simulink model "vschvdc"  (R2023a)
settings: Solver=ode45  StartTime=0.0  StopTime=10.0  RelTol=1e-3
InitFcn:
  | P=1e6;
  | V=6e3;
  | F=50;
  | 
  | VDC=6e3;
  | C=200e-6;
  | 
  | R=1e-3;
  | L=0.1;
  | Ts_control=50e-6;
  | Ts=1e-6;
undefined symbols (not defined in the file): D1, Delta, DiscIntNeverNeededParam, init, Ki, Kp, LOW, UP
libraries: spsThreePhaseVIMeasurementLib x6, spsGroundLib x2, spsabctodq0Lib x2, spsThreePhaseSeriesRLCBranchLib x2, spsThreePhaseSeriesRLCLoadLib x2, spsThreePhaseTransformerTwoWindingsLib x2, spsSeriesRLCBranchLib x2, spsUniversalBridgeLib x2, spsVoltageMeasurementLib x2, spsPiSectionLineLib x2, spsThreePhaseMutualInductanceZ1Z0Lib x2, spsThreePhaseProgrammableVoltageSourceLib x2
settings Model: Creator=11094  LastModifiedBy=11094

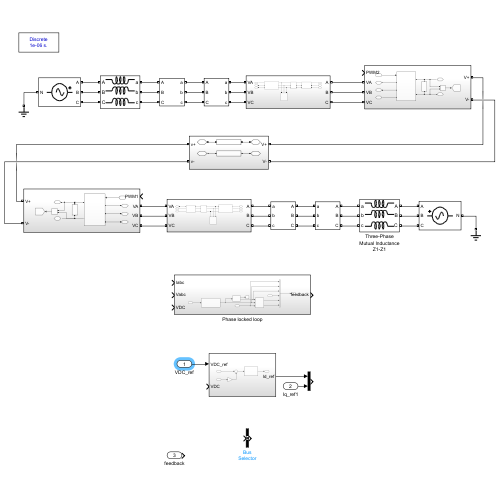
[thumbnail: Simulink's stored preview of the top-level diagram]
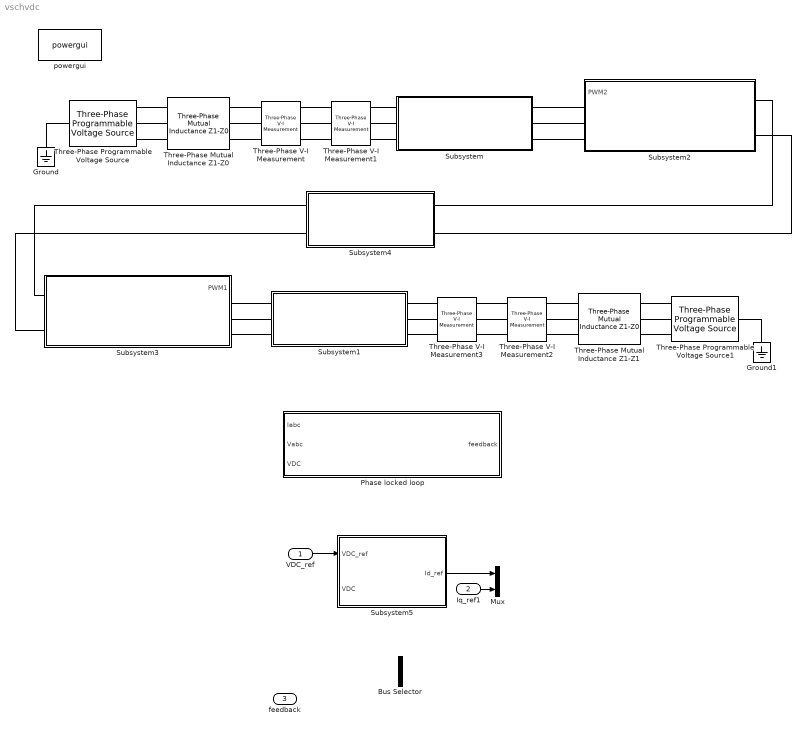
== system vschvdc ==
  VDC_ref : Inport
  Iq_ref1 : Inport  Port=2
  feedback : Inport  Port=3
  Bus Selector : BusSelector  OutputSignals=signal1
  Ground : spsGroundLib/Ground  LConnTagsString=a
  Ground1 : spsGroundLib/Ground  LConnTagsString=a
  Mux : Mux  Inputs=2
  Phase locked loop : Subsystem
  Subsystem : Subsystem
  Subsystem1 : Subsystem
  Subsystem2 : Subsystem
  Subsystem3 : Subsystem
  Subsystem4 : Subsystem
  Subsystem5 : Subsystem
  Three-Phase Mutual Inductance Z1-Z0 : spsThreePhaseMutualInductanceZ1Z0Lib/Three-Phase Mutual Inductance Z1-Z0  LConnTagsString=a|b|c  RConnTagsString=A|B|C  PositiveSequence="[ 220e3^2/(10*P)/10  220e3^2/(10*P)/(2*pi*50)]"  ZeroSequence="[ 220e3^2/(10*P)/10*3  220e3^2/(10*P)/(2*pi*50)*3]"
      settings: AttributesFormatString=\n
      settings: LibrarySourceBlock=|
      | sps_lib/Power Grid Elements/Three-Phase
      | Mutual Inductance
      | Z1-Z0
  Three-Phase Mutual Inductance Z1-Z1 : spsThreePhaseMutualInductanceZ1Z0Lib/Three-Phase Mutual Inductance Z1-Z0  LConnTagsString=a|b|c  RConnTagsString=A|B|C  PositiveSequence="[ 220e3^2/(10*P)/10  220e3^2/(10*P)/(2*pi*50)]"  ZeroSequence="[ 220e3^2/(10*P)/10*3  220e3^2/(10*P)/(2*pi*50)*3]"
      settings: AttributesFormatString=\n
      settings: LibrarySourceBlock=|
      | sps_lib/Power Grid Elements/Three-Phase
      | Mutual Inductance
      | Z1-Z0
  Three-Phase Programmable Voltage Source : spsThreePhaseProgrammableVoltageSourceLib/Three-Phase Programmable Voltage Source  PositiveSequence="[220e3  0 50]"  VariationEntity=None  VariationType=Table of time-amplitude pairs  VariationTypeAlt=Step  VariationStep=0.5  VariationRate=10  VariationMagnitude=0.3  VariationFrequency=2  VariationTiming=[1 2]  VariationPhaseA=off  Amplitudes=[1 0.8 1.2 1.0]  TimeValues=[0 0.1 0.15 0.2]  HarmonicGeneration=off  HarmonicA=[3 0.2 -25 0]  HarmonicB=[2 0.15 35 2]  Timing="[0.05  3]"  BusType=swing  Pref=0  Qref=0  Qmin=-inf  Qmax=inf
  Three-Phase Programmable Voltage Source1 : spsThreePhaseProgrammableVoltageSourceLib/Three-Phase Programmable Voltage Source  PositiveSequence="[220e3  0 50]"  VariationEntity=None  VariationType=Table of time-amplitude pairs  VariationTypeAlt=Step  VariationStep=0.5  VariationRate=10  VariationMagnitude=0.3  VariationFrequency=2  VariationTiming=[1 2]  VariationPhaseA=off  Amplitudes=[1 0.8 1.2 1.0]  TimeValues=[0 0.1 0.15 0.2]  HarmonicGeneration=off  HarmonicA=[3 0.2 -25 0]  HarmonicB=[2 0.15 35 2]  Timing="[0.05  3]"  BusType=swing  Pref=0  Qref=0  Qmin=-inf  Qmax=inf
  Three-Phase V-I Measurement : spsThreePhaseVIMeasurementLib/Three-Phase V-I Measurement  VoltageMeasurement=phase-to-phase  SetLabelV=on  LabelV=Vabc2  Vpu=off  VpuLL=off  CurrentMeasurement=yes  SetLabelI=on  LabelI=Iabc2  Ipu=off  Pbase=100e6  Vbase=500e3  OutputType=Complex  PhasorSimulation=off  PSBequivalent=0
  Three-Phase V-I Measurement1 : spsThreePhaseVIMeasurementLib/Three-Phase V-I Measurement  VoltageMeasurement=phase-to-phase  SetLabelV=on  LabelV=Vabc_B3  Vpu=off  VpuLL=on  CurrentMeasurement=yes  SetLabelI=on  LabelI=Iabc_B3  Ipu=on  Pbase=P  Vbase=V  OutputType=Complex  PhasorSimulation=off  PSBequivalent=0
  Three-Phase V-I Measurement2 : spsThreePhaseVIMeasurementLib/Three-Phase V-I Measurement  VoltageMeasurement=phase-to-phase  SetLabelV=on  LabelV=Vabc1  Vpu=off  VpuLL=off  CurrentMeasurement=yes  SetLabelI=on  LabelI=Iabc1  Ipu=off  Pbase=100e6  Vbase=500e3  OutputType=Complex  PhasorSimulation=off  PSBequivalent=0
  Three-Phase V-I Measurement3 : spsThreePhaseVIMeasurementLib/Three-Phase V-I Measurement  VoltageMeasurement=phase-to-phase  SetLabelV=on  LabelV=Vabc_B1  Vpu=off  VpuLL=on  CurrentMeasurement=yes  SetLabelI=on  LabelI=Iabc_B1  Ipu=on  Pbase=P  Vbase=V  OutputType=Complex  PhasorSimulation=off  PSBequivalent=0
  powergui : spspowerguiLib/powergui  Priority=1  SimulationMode=Discrete  SampleTime=1e-6  frequency=60  Iterations=50  frequencyindice=60  Pbase=100e6  ErrMax=1e-4  UnitsV=kV  UnitsW=MW  buscounter=0  FunctionMessages=off  echomessages=off  EnableUseOfTLC=off  CurrentSourceSwitches=off  DisableSnubberDevices=off  DisableRonSwitches=off  DisableVfSwitches=off  DisplayEquations=off  AutomaticDiscreteSolvers=off  SolverType=Tustin/Backward Euler (TBE)  Interpol=off  ExternalGateDelay=off  methode=off  Ts=100  x0status=blocks  SPID=on  SwTol=0  HookPort=off  NonlinearTolerance=1e-4  nMaxIteration=100  ContinueOnMaxIteration=off  RestoreLinks=warning  ResistiveCurrentMeasurement=off  Frange=[0:2:500]  Ylog=off  Xlog=on  ShowGrid=off  save=off  variable=ZData  structure=0  ZoomFFT=off  StartTime=0.0  cycles=1  DisplayStyle=1  fundamental=60  FreqAxis=off  MaxFrequency=1000  frequencyindicesteady=1  RmsSteady=1  display=off
  wires:
  Subsystem5/1(Id_ref) -> Mux/1
  Iq_ref1/1 -> Mux/2
  VDC_ref/1 -> Subsystem5/1(VDC_ref)
  connections:
  Three-Phase Programmable Voltage Source/LConn1 -- Ground/LConn1
  Three-Phase Mutual Inductance Z1-Z0/LConn2 -- Three-Phase Programmable Voltage Source/RConn2
  Three-Phase Mutual Inductance Z1-Z0/LConn3 -- Three-Phase Programmable Voltage Source/RConn3
  Three-Phase Mutual Inductance Z1-Z0/LConn1 -- Three-Phase Programmable Voltage Source/RConn1
  Three-Phase V-I Measurement/LConn1 -- Three-Phase Mutual Inductance Z1-Z0/RConn1
  Three-Phase V-I Measurement/LConn2 -- Three-Phase Mutual Inductance Z1-Z0/RConn2
  Three-Phase V-I Measurement/LConn3 -- Three-Phase Mutual Inductance Z1-Z0/RConn3
  Three-Phase V-I Measurement/RConn1 -- Three-Phase V-I Measurement1/LConn1
  Three-Phase V-I Measurement/RConn2 -- Three-Phase V-I Measurement1/LConn2
  Three-Phase V-I Measurement/RConn3 -- Three-Phase V-I Measurement1/LConn3
  Subsystem/LConn1 -- Three-Phase V-I Measurement1/RConn1
  Subsystem/LConn2 -- Three-Phase V-I Measurement1/RConn2
  Subsystem/LConn3 -- Three-Phase V-I Measurement1/RConn3
  Three-Phase Mutual Inductance Z1-Z1/LConn1 -- Three-Phase Programmable Voltage Source1/RConn1
  Three-Phase V-I Measurement2/LConn2 -- Three-Phase Mutual Inductance Z1-Z1/RConn2
  Three-Phase Mutual Inductance Z1-Z1/LConn3 -- Three-Phase Programmable Voltage Source1/RConn3
  Three-Phase V-I Measurement2/LConn1 -- Three-Phase Mutual Inductance Z1-Z1/RConn1
  Three-Phase V-I Measurement2/RConn2 -- Three-Phase V-I Measurement3/LConn2
  Three-Phase Mutual Inductance Z1-Z1/LConn2 -- Three-Phase Programmable Voltage Source1/RConn2
  Three-Phase V-I Measurement2/LConn3 -- Three-Phase Mutual Inductance Z1-Z1/RConn3
  Three-Phase Programmable Voltage Source1/LConn1 -- Ground1/LConn1
  Three-Phase V-I Measurement2/RConn3 -- Three-Phase V-I Measurement3/LConn3
  Three-Phase V-I Measurement2/RConn1 -- Three-Phase V-I Measurement3/LConn1
  Subsystem1/RConn1 -- Three-Phase V-I Measurement3/RConn1
  Subsystem1/RConn2 -- Three-Phase V-I Measurement3/RConn2
  Subsystem1/RConn3 -- Three-Phase V-I Measurement3/RConn3
  Subsystem2/LConn3 -- Subsystem/RConn3
  Subsystem/RConn2 -- Subsystem2/LConn2
  Subsystem/RConn1 -- Subsystem2/LConn1
  Subsystem3/LConn3 -- Subsystem1/LConn3
  Subsystem3/LConn2 -- Subsystem1/LConn2
  Subsystem3/LConn1 -- Subsystem1/LConn1
  Subsystem4/RConn1 -- Subsystem3/RConn1
  Subsystem4/RConn2 -- Subsystem3/RConn2
  Subsystem2/RConn1 -- Subsystem4/LConn1
  Subsystem2/RConn2 -- Subsystem4/LConn2

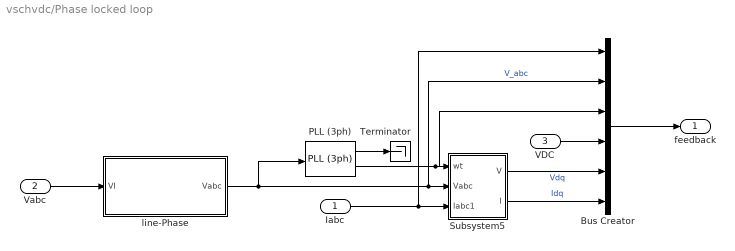
== system vschvdc/Phase locked loop ==
  Iabc : Inport
  Vabc : Inport  Port=2
  VDC : Inport  Port=3
  Bus Creator : BusCreator  Inputs=6
  PLL (3ph) : spsPLL3phLib/PLL (3ph)  Fmin=45  Par_Init=[0, F]  ParK=[60, 1400]  TcD=0.04  MaxRateChangeFreq=12  FilterCutOffFreq=25  Ts=Ts  AGC=on
  Subsystem5 : Subsystem
  Terminator : Terminator
  line-Phase : Subsystem
  feedback : Outport
  wires:
  Bus Creator/1 -> feedback/1
  Iabc/1 -> Bus Creator/1, Subsystem5/3(Iabc1)
  PLL (3ph)/2 -> Bus Creator/3, Subsystem5/1(wt)
  Subsystem5/1(V) -> Bus Creator/5  "Vdq"
  PLL (3ph)/1 -> Terminator/1
  line-Phase/1(Vabc) -> PLL (3ph)/1, Bus Creator/2, Subsystem5/2(Vabc)  "V_abc"
  Vabc/1 -> line-Phase/1(VI)
  Subsystem5/2(I) -> Bus Creator/6  "Idq"
  VDC/1 -> Bus Creator/4

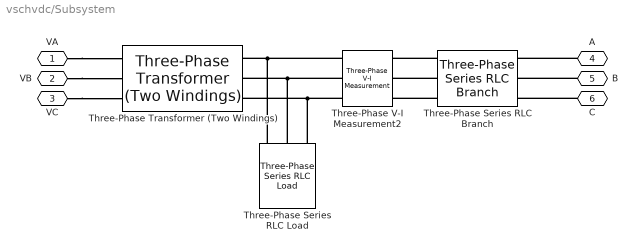
== system vschvdc/Subsystem ==
  Three-Phase Series RLC Branch : spsThreePhaseSeriesRLCBranchLib/Three-Phase Series RLC Branch  LConnTagsString=A|B|C  RConnTagsString=A|B|C  BranchType=RL  Resistance=R*V^2/P  Inductance=L*V^2/P/(2*pi*F)  Capacitance=1e-6  Measurements=None
  Three-Phase Series RLC Load : spsThreePhaseSeriesRLCLoadLib/Three-Phase Series RLC Load  LConnTagsString=A|B|C  Configuration=Y (grounded)  NominalVoltage=V  Vabc=[1e3 1e3 1e3]  Vabcp=[1e3 1e3 1e3]  NominalFrequency=F  UnbalancedPower=off  ActivePower=P*0.1/50  InductivePower=0  CapacitivePower=P*0.15  Pabc=[10e3 9e3 11e3]  QLabc=[100 90 110]  QCabc=[100 90 110]  Pabcp=[10e3 9e3 11e3]  QLabcp=[100 90 110]  QCabcp=[100 90 110]  Measurements=None  LoadType=constant Z
  Three-Phase Transformer (Two Windings) : spsThreePhaseTransformerTwoWindingsLib/Three-Phase Transformer (Two Windings)  Winding1Connection=Yg  Winding2Connection=Delta (D1)  CoreType=Three single-phase transformers  SetSaturation=off  Hysteresis=off  DataFile='hysteresis'  SetInitialFlux=off  Measurements=None  UNITS=pu  NominalPower=[ P*1.5 , 50 ]  Winding1=[ 220e3 , 0.5/30 , 0.05 ]  Winding2=[ V , 0.05/30 , 0.05 ]  Rm=500  Lm=500  L0=0.5  Saturation=[ 0,0 ; 0.0024,1.2 ; 1.0,1.52 ]  InitialFluxes=[ 0.8 , -0.8 , 0.7 ]  BreakLoop=off  DiscreteSolver=Trapezoidal iterative  DataType=off  TransfoNumber=1
  Three-Phase V-I Measurement2 : spsThreePhaseVIMeasurementLib/Three-Phase V-I Measurement  VoltageMeasurement=phase-to-phase  SetLabelV=on  LabelV=Vabc_B4  Vpu=off  VpuLL=on  CurrentMeasurement=yes  SetLabelI=on  LabelI=Iabc_B4  Ipu=on  Pbase=P  Vbase=V  OutputType=Complex  PhasorSimulation=off  PSBequivalent=0
  VA : PMIOPort  Side=Left
  VB : PMIOPort  Port=2  Side=Left
  VC : PMIOPort  Port=3  Side=Left
  A : PMIOPort  Port=4  Side=Right
  B : PMIOPort  Port=5  Side=Right
  C : PMIOPort  Port=6  Side=Right
  connections:
  A/RConn1 -- Three-Phase Series RLC Branch/RConn1
  Three-Phase V-I Measurement2/LConn3 -- Three-Phase Series RLC Load/LConn3 -- Three-Phase Transformer (Two Windings)/RConn3
  VB/RConn1 -- Three-Phase Transformer (Two Windings)/LConn2
  C/RConn1 -- Three-Phase Series RLC Branch/RConn3
  VA/RConn1 -- Three-Phase Transformer (Two Windings)/LConn1
  Three-Phase V-I Measurement2/LConn1 -- Three-Phase Series RLC Load/LConn1 -- Three-Phase Transformer (Two Windings)/RConn1
  Three-Phase V-I Measurement2/LConn2 -- Three-Phase Series RLC Load/LConn2 -- Three-Phase Transformer (Two Windings)/RConn2
  Three-Phase Series RLC Branch/LConn3 -- Three-Phase V-I Measurement2/RConn3
  B/RConn1 -- Three-Phase Series RLC Branch/RConn2
  Three-Phase Series RLC Branch/LConn1 -- Three-Phase V-I Measurement2/RConn1
  VC/RConn1 -- Three-Phase Transformer (Two Windings)/LConn3
  Three-Phase Series RLC Branch/LConn2 -- Three-Phase V-I Measurement2/RConn2

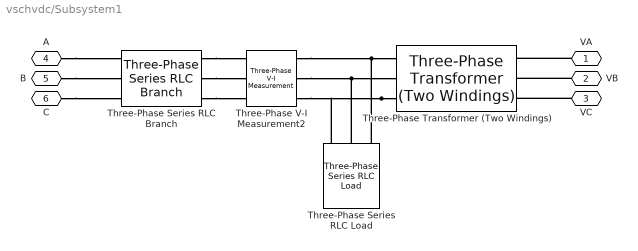
== system vschvdc/Subsystem1 ==
  Three-Phase Series RLC Branch : spsThreePhaseSeriesRLCBranchLib/Three-Phase Series RLC Branch  LConnTagsString=A|B|C  RConnTagsString=A|B|C  BranchType=RL  Resistance=R*V^2/P  Inductance=L*V^2/P/(2*pi*F)  Capacitance=1e-6  Measurements=None
  Three-Phase Series RLC Load : spsThreePhaseSeriesRLCLoadLib/Three-Phase Series RLC Load  LConnTagsString=A|B|C  Configuration=Y (grounded)  NominalVoltage=V  Vabc=[1e3 1e3 1e3]  Vabcp=[1e3 1e3 1e3]  NominalFrequency=F  UnbalancedPower=off  ActivePower=P*0.1/50  InductivePower=0  CapacitivePower=P*0.15  Pabc=[10e3 9e3 11e3]  QLabc=[100 90 110]  QCabc=[100 90 110]  Pabcp=[10e3 9e3 11e3]  QLabcp=[100 90 110]  QCabcp=[100 90 110]  Measurements=None  LoadType=constant Z
  Three-Phase Transformer (Two Windings) : spsThreePhaseTransformerTwoWindingsLib/Three-Phase Transformer (Two Windings)  Winding1Connection=Yg  Winding2Connection=Delta (D1)  CoreType=Three single-phase transformers  SetSaturation=off  Hysteresis=off  DataFile='hysteresis'  SetInitialFlux=off  Measurements=None  UNITS=pu  NominalPower=[ P*1.5 , 50 ]  Winding1=[ 220e3 , 0.5/30 , 0.05 ]  Winding2=[ V , 0.05/30 , 0.05 ]  Rm=500  Lm=500  L0=0.5  Saturation=[ 0,0 ; 0.0024,1.2 ; 1.0,1.52 ]  InitialFluxes=[ 0.8 , -0.8 , 0.7 ]  BreakLoop=off  DiscreteSolver=Trapezoidal iterative  DataType=off  TransfoNumber=1
  Three-Phase V-I Measurement2 : spsThreePhaseVIMeasurementLib/Three-Phase V-I Measurement  VoltageMeasurement=phase-to-phase  SetLabelV=on  LabelV=Vabc_B2  Vpu=off  VpuLL=on  CurrentMeasurement=yes  SetLabelI=on  LabelI=Iabc_B2  Ipu=on  Pbase=P  Vbase=V  OutputType=Complex  PhasorSimulation=off  PSBequivalent=0
  VA : PMIOPort  Side=Left
  VB : PMIOPort  Port=2  Side=Left
  VC : PMIOPort  Port=3  Side=Left
  A : PMIOPort  Port=4  Side=Right
  B : PMIOPort  Port=5  Side=Right
  C : PMIOPort  Port=6  Side=Right
  connections:
  A/RConn1 -- Three-Phase Series RLC Branch/RConn1
  Three-Phase Transformer (Two Windings)/RConn3 -- Three-Phase Series RLC Load/LConn3 -- Three-Phase V-I Measurement2/LConn3
  VB/RConn1 -- Three-Phase Transformer (Two Windings)/LConn2
  C/RConn1 -- Three-Phase Series RLC Branch/RConn3
  VA/RConn1 -- Three-Phase Transformer (Two Windings)/LConn1
  Three-Phase V-I Measurement2/LConn1 -- Three-Phase Series RLC Load/LConn1 -- Three-Phase Transformer (Two Windings)/RConn1
  Three-Phase V-I Measurement2/LConn2 -- Three-Phase Series RLC Load/LConn2 -- Three-Phase Transformer (Two Windings)/RConn2
  Three-Phase Series RLC Branch/LConn3 -- Three-Phase V-I Measurement2/RConn3
  B/RConn1 -- Three-Phase Series RLC Branch/RConn2
  Three-Phase Series RLC Branch/LConn1 -- Three-Phase V-I Measurement2/RConn1
  VC/RConn1 -- Three-Phase Transformer (Two Windings)/LConn3
  Three-Phase Series RLC Branch/LConn2 -- Three-Phase V-I Measurement2/RConn2

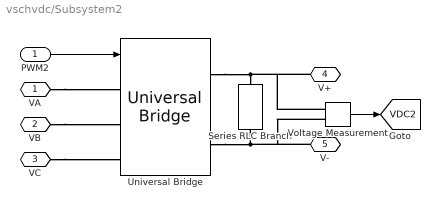
== system vschvdc/Subsystem2 ==
  PWM2 : Inport
  Series RLC Branch : spsSeriesRLCBranchLib/Series RLC Branch  LConnTagsString=__new0  RConnTagsString=__new0  BranchType=C  Resistance=1  Inductance=1e-3  SetiL0=off  InitialCurrent=0  Capacitance=C  Setx0=on  InitialVoltage=VDC  Measurements=None
  Universal Bridge : spsUniversalBridgeLib/Universal Bridge  Arms=3  SnubberResistance=5000  SnubberCapacitance=1e-6  Device=IGBT / Diodes  Ron=1e-3  Lon=0  ForwardVoltages="[  0  0  ]"  ForwardVoltage=0  GTOparameters=[ 10e-6 , 20e-6 ]  IGBTparameters=[ 1e-6 , 2e-6 ]  Measurements=None  Measurements_2=None  converterType=Rectifier
  Voltage Measurement : spsVoltageMeasurementLib/Voltage Measurement  PhasorSimulation=off  OutputType=Complex  PSBequivalent=0
  VA : PMIOPort  Side=Left
  VB : PMIOPort  Port=2  Side=Left
  VC : PMIOPort  Port=3  Side=Left
  V+ : PMIOPort  Port=4  Side=Right
  V- : PMIOPort  Port=5  Side=Right
  tag scope: VDC2=global
  wires:
  PWM2/1 -> Universal Bridge/1
  Voltage Measurement/1 -> [VDC2]
  connections:
  VA/RConn1 -- Universal Bridge/LConn1
  VC/RConn1 -- Universal Bridge/LConn3
  VB/RConn1 -- Universal Bridge/LConn2
  Universal Bridge/RConn2 -- V-/RConn1 -- Voltage Measurement/LConn2 -- Series RLC Branch/RConn1
  Universal Bridge/RConn1 -- V+/RConn1 -- Voltage Measurement/LConn1 -- Series RLC Branch/LConn1

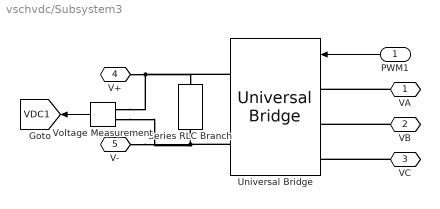
== system vschvdc/Subsystem3 ==
  PWM1 : Inport
  Series RLC Branch : spsSeriesRLCBranchLib/Series RLC Branch  LConnTagsString=__new0  RConnTagsString=__new0  BranchType=C  Resistance=1  Inductance=1e-3  SetiL0=off  InitialCurrent=0  Capacitance=C  Setx0=on  InitialVoltage=VDC  Measurements=None
  Universal Bridge : spsUniversalBridgeLib/Universal Bridge  Arms=3  SnubberResistance=5000  SnubberCapacitance=1e-6  Device=IGBT / Diodes  Ron=1e-3  Lon=0  ForwardVoltages="[  0  0  ]"  ForwardVoltage=0  GTOparameters=[ 10e-6 , 20e-6 ]  IGBTparameters=[ 1e-6 , 2e-6 ]  Measurements=None  Measurements_2=None  converterType=Rectifier
  Voltage Measurement : spsVoltageMeasurementLib/Voltage Measurement  PhasorSimulation=off  OutputType=Complex  PSBequivalent=0
  VA : PMIOPort  Side=Left
  VB : PMIOPort  Port=2  Side=Left
  VC : PMIOPort  Port=3  Side=Left
  V+ : PMIOPort  Port=4  Side=Right
  V- : PMIOPort  Port=5  Side=Right
  tag scope: VDC1=global
  wires:
  PWM1/1 -> Universal Bridge/1
  Voltage Measurement/1 -> [VDC1]
  connections:
  VA/RConn1 -- Universal Bridge/LConn1
  VC/RConn1 -- Universal Bridge/LConn3
  VB/RConn1 -- Universal Bridge/LConn2
  Voltage Measurement/LConn2 -- Series RLC Branch/RConn1 -- Universal Bridge/RConn2 -- V-/RConn1
  Voltage Measurement/LConn1 -- Universal Bridge/RConn1 -- Series RLC Branch/LConn1 -- V+/RConn1

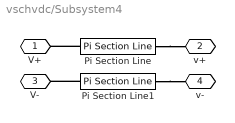
== system vschvdc/Subsystem4 ==
  Pi Section Line : spsPiSectionLineLib/Pi Section Line  LConnTagsString=1  RConnTagsString=1  Phases=1  PiSections=1  Length=100  Frequency=50  Resistance=1.031e-3  Inductance=1.05e-4  Capacitance=2.1e-7  SpecifyConductance=off  Conductance=0  Measurements=None  Measurements2=None
      settings: LibrarySourceBlock=sps_lib/Power Grid Elements/Pi Section Line
  Pi Section Line1 : spsPiSectionLineLib/Pi Section Line  LConnTagsString=1  RConnTagsString=1  Phases=1  PiSections=1  Length=100  Frequency=50  Resistance=1.031e-3  Inductance=1.05e-4  Capacitance=2.1e-7  SpecifyConductance=off  Conductance=0  Measurements=None  Measurements2=None
      settings: LibrarySourceBlock=sps_lib/Power Grid Elements/Pi Section Line
  V+ : PMIOPort  Side=Left
  v+ : PMIOPort  Port=2  Side=Right
  V- : PMIOPort  Port=3  Side=Left
  v- : PMIOPort  Port=4  Side=Right
  connections:
  Pi Section Line1/RConn1 -- v-/RConn1
  Pi Section Line1/LConn1 -- V-/RConn1
  Pi Section Line/RConn1 -- v+/RConn1
  Pi Section Line/LConn1 -- V+/RConn1

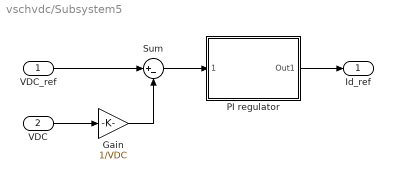
== system vschvdc/Subsystem5 ==
  VDC_ref : Inport
  VDC : Inport  Port=2
  Gain : Gain  Gain=1/VDC
  PI regulator : Subsystem
      mask DialogControl ParameterGroupVar Prompt: 参数
  Sum : Sum  Inputs=|+-
  Id_ref : Outport
  wires:
  Sum/1 -> PI regulator/1(" ")
  Gain/1 -> Sum/2
  VDC/1 -> Gain/1
  PI regulator/1(Out1) -> Id_ref/1
  VDC_ref/1 -> Sum/1

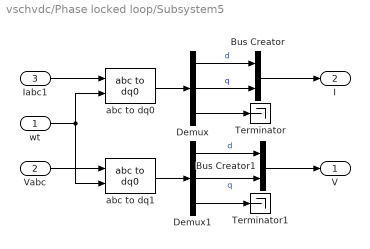
== system vschvdc/Phase locked loop/Subsystem5 ==
  wt : Inport
  Vabc : Inport  Port=2
  Iabc1 : Inport  Port=3
  Bus Creator : BusCreator  Inputs=2
  Bus Creator1 : BusCreator  Inputs=2
  Demux : Demux  Outputs=3
  Demux1 : Demux  Outputs=3
  Terminator : Terminator
  Terminator1 : Terminator
  abc to dq0 : spsabctodq0Lib/abc to dq0  Alignment=90 degrees behind phase A axis
  abc to dq1 : spsabctodq0Lib/abc to dq0  Alignment=90 degrees behind phase A axis
  V : Outport
  I : Outport  Port=2
  wires:
  wt/1 -> abc to dq1/2, abc to dq0/2
  Demux/3 -> Terminator/1
  Bus Creator/1 -> I/1
  Demux1/2 -> Bus Creator1/2  "q"
  Demux/1 -> Bus Creator/1  "d"
  Demux1/1 -> Bus Creator1/1  "d"
  Demux/2 -> Bus Creator/2  "q"
  abc to dq1/1 -> Demux1/1
  abc to dq0/1 -> Demux/1
  Iabc1/1 -> abc to dq0/1
  Vabc/1 -> abc to dq1/1
  Demux1/3 -> Terminator1/1
  Bus Creator1/1 -> V/1

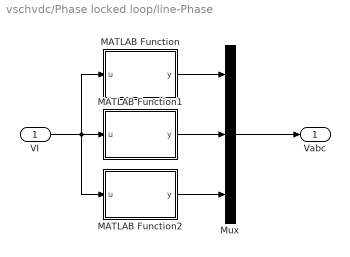
== system vschvdc/Phase locked loop/line-Phase ==
  VI : Inport
  MATLAB Function : MATLAB Function  TreatAsAtomicUnit=on
  MATLAB Function1 : MATLAB Function  TreatAsAtomicUnit=on
  MATLAB Function2 : MATLAB Function  TreatAsAtomicUnit=on
  Mux : Mux  Inputs=3
  Vabc : Outport
  wires:
  MATLAB Function1/1(y) -> Mux/2
  VI/1 -> MATLAB Function2/1(u), MATLAB Function/1(u), MATLAB Function1/1(u)
  Mux/1 -> Vabc/1
  MATLAB Function/1(y) -> Mux/1
  MATLAB Function2/1(y) -> Mux/3

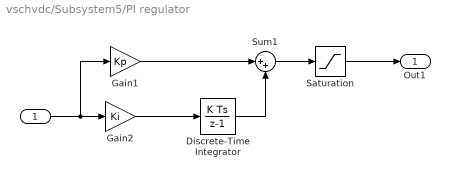
== system vschvdc/Subsystem5/PI regulator ==
  " " : Inport
  Discrete-Time Integrator : DiscreteIntegrator  InitialCondition=init  SampleTime=Ts  LimitOutput=on  UpperSaturationLimit=UP  LowerSaturationLimit=LOW  ICPrevOutput=DiscIntNeverNeededParam  ICPrevScaledInput=DiscIntNeverNeededParam
  Gain1 : Gain  Gain=Kp
  Gain2 : Gain  Gain=Ki
  Saturation : Saturate  UpperLimit=UP  LowerLimit=LOW
  Sum1 : Sum  Inputs=|++
  Out1 : Outport
  wires:
  Sum1/1 -> Saturation/1
  Discrete-Time Integrator/1 -> Sum1/2
  " "/1 -> Gain1/1, Gain2/1
  Gain1/1 -> Sum1/1
  Gain2/1 -> Discrete-Time Integrator/1
  Saturation/1 -> Out1/1

== matlab function vschvdc/Phase locked loop/line-Phase/MATLAB Function ==
  data: u input; y output
function y = fcn(u)

y = (u(1)-u(3))/3;

== matlab function vschvdc/Phase locked loop/line-Phase/MATLAB Function2 ==
  data: u input; y output
function y = fcn(u)

y = (u(3)-u(2))/3;

== matlab function vschvdc/Phase locked loop/line-Phase/MATLAB Function1 ==
  data: u input; y output
function y = fcn(u)

y = (u(2)-u(1))/3;
